simulink model "prob1"  (R2020a)
settings: Solver=VariableStepAuto  StartTime=0.0  StopTime=10.0  RelTol=1e-3
settings Model: Creator=vijay  LastModifiedBy=vijay

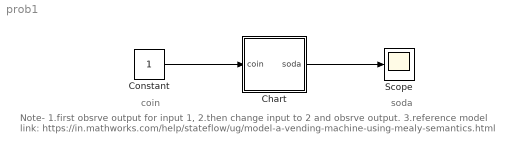
== system prob1 ==
  note: soda
  note: coin
  note: Note-
      |
      | 1.first obsrve output for input 1,
      | 2.then change input to 2 and obsrve output.
      | 3.reference model link:
      | https://in.mathworks.com/help/stateflow/ug/model-a-vending-machine-using-mealy-semantics.html
  Chart : Stateflow chart  TreatAsAtomicUnit=on
  Constant : Constant
  Scope : Scope
  wires:
  Constant/1 -> Chart/1(coin)
  Chart/1(soda) -> Scope/1

== stateflow chart prob1/Chart ==
  state got0
  state gotn
  state gotd
  (default) -> got0
  got0 -> gotn [order 1] : [coin==1]{soda=0}
  gotn -> got0 [order 1] : [coin==2]{soda=1}
  gotd -> got0 [order 2] : [coin==1]{soda=1}
  got0 -> gotd [order 2] : [coin==2]{soda=0}
  gotn -> gotd [order 2] : [coin==1]{soda=0}
  gotd -> gotn [order 1] : [coin==2]{soda=1}
  data: coin input; soda output
